simulink model "ultrasonic_parking_assist"  (R2024a)
settings: Solver=VariableStepAuto  StartTime=0.0  StopTime=7.5  RelTol=1e-3
libraries: simulink x1
settings Model: Creator=chiemerieokeke  LastModifiedBy=chiemerieokeke

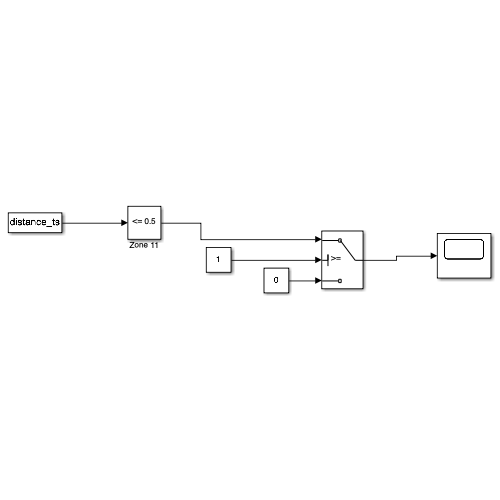
[thumbnail: Simulink's stored preview of the top-level diagram]
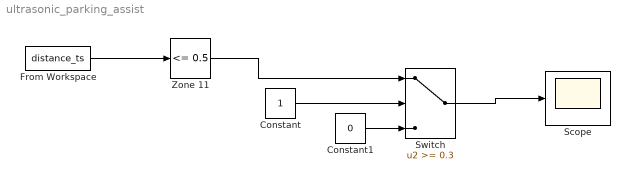
== system ultrasonic_parking_assist ==
  Constant : Constant
  Constant1 : Constant  Value=0
  From Workspace : FromWorkspace  VariableName=distance_ts  SampleTime=-1
  Scope : Scope
  Switch : Switch  Threshold=0.3  SaturateOnIntegerOverflow=off  InputSameDT=off
  Zone 11 : simulink/Logic and Bit Operations/Compare To Constant  relop=<=  const=0.5  OutDataTypeStr=boolean
  wires:
  Constant1/1 -> Switch/3
  Constant/1 -> Switch/2
  Zone 11/1 -> Switch/1
  From Workspace/1 -> Zone 11/1
  Switch/1 -> Scope/1
